simulink model "jav1"  (R2025b)
settings: Solver=VariableStepAuto  StartTime=0.0  StopTime=10.0  RelTol=1e-3
undefined symbols (not defined in the file): delta_pitch_saturation, g, I_treghet, K_drag, K_finne, Kd_pitch, Ki_altitude, Kp_altitude, Kp_pitch, L_aksial, m, T, theta0, theta_dot, theta_ff, theta_ref_saturation, v_x0, v_z0, x0, z0, z_ref
libraries: slpidlib x1
settings Model: Creator=Tobias Stenberg  LastModifiedBy=Tobias Stenberg

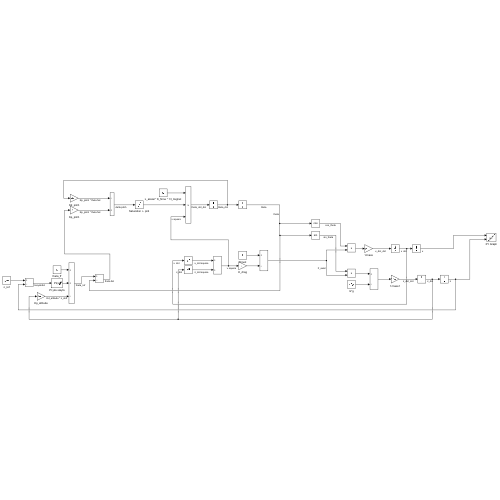
[thumbnail: Simulink's stored preview of the top-level diagram]
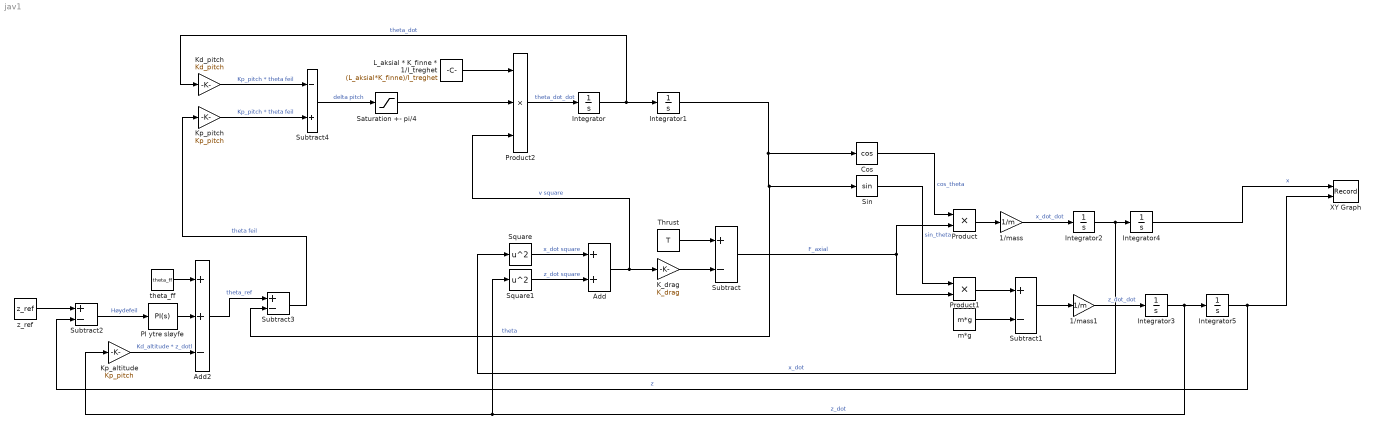
== system jav1 ==
  1/mass : Gain  Gain=1/m
  1/mass1 : Gain  Gain=1/m
  Add : Sum
  Add2 : Sum  Inputs=++-
  Cos : Trigonometry  Operator=cos
  Integrator : Integrator  InitialCondition=theta_dot
  Integrator1 : Integrator  InitialCondition=theta0
  Integrator2 : Integrator  InitialCondition=v_x0
  Integrator3 : Integrator  InitialCondition=v_z0
  Integrator4 : Integrator  InitialCondition=x0
  Integrator5 : Integrator  InitialCondition=z0
  K_drag : Gain  Gain=K_drag
  Kd_pitch : Gain  Gain=Kd_pitch
  Kp_altitude : Gain  Gain=Kp_pitch
  Kp_pitch : Gain  Gain=Kp_pitch
  L_aksial * K_finne * 1/I_treghet : Constant  Value=(L_aksial*K_finne)/I_treghet
  PI ytre sløyfe : slpidlib/PID Controller  Controller=PI  Form=Parallel  TimeDomain=Continuous-time  UseExternalTs=off  SampleTime=-1  IntegratorMethod=Forward Euler  FilterMethod=Forward Euler  ControllerParametersSource=internal  P=Kp_altitude  I=Ki_altitude  UseKiTs=off  D=0  UseExternalDerivativeSource=off  N=100  UseFilter=on  TunerSelectOption=Transfer Function Based (PID Tuner App)  ZeroCross=off  InitialConditionSource=internal  InitialConditionForIntegrator=0  InitialConditionForFilter=0  DifferentiatorICPrevScaledInput=0  ExternalReset=none  TrackingMode=off  Kt=1  LimitOutput=on  SatLimitsSource=internal  UpperSaturationLimit=theta_ref_saturation  LowerSaturationLimit=-theta_ref_saturation  LinearizeAsGain=on  AntiWindupMode=clamping  Kb=1  LimitIntegrator=off  UpperIntegratorSaturationLimit=inf  LowerIntegratorSaturationLimit=-inf  POutMin=[]  POutMax=[]  IOutMin=[]  IOutMax=[]  DOutMin=[]  DOutMax=[]  NOutMin=[]  NOutMax=[]  SumOutMin=[]  SumOutMax=[]  SaturationOutMin=[]  SaturationOutMax=[]  PParamMin=[]  PParamMax=[]  IParamMin=[]  IParamMax=[]  DParamMin=[]  DParamMax=[]  NParamMin=[]  NParamMax=[]  KbParamMin=[]  KbParamMax=[]  KtParamMin=[]  KtParamMax=[]  KbOutMin=[]  KbOutMax=[]  KtOutMin=[]  KtOutMax=[]  IntegratorOutMin=[]  IntegratorOutMax=[]  FilterOutMin=[]  FilterOutMax=[]  SumI1OutMin=[]  SumI1OutMax=[]  SumI2OutMin=[]  SumI2OutMax=[]  SumI3OutMin=[]  SumI3OutMax=[]  SumI4OutMin=[]  SumI4OutMax=[]  SumDOutMin=[]  SumDOutMax=[]  DifferentiatorOutMin=[]  DifferentiatorOutMax=[]  FilterDiffOutCoefMin=[]  FilterDiffOutCoefMax=[]  ReciprocalOutMin=[]  ReciprocalOutMax=[]  SumDenOutMin=[]  SumDenOutMax=[]  SumNumOutMin=[]  SumNumOutMax=[]  DivideOutMin=[]  DivideOutMax=[]  UdiffTsProdOutMin=[]  UdiffTsProdOutMax=[]  NTsProdOutMin=[]  NTsProdOutMax=[]  UintegralTsProdOutMin=[]  UintegralTsProdOutMax=[]  UngainTsProdOutMin=[]  UngainTsProdOutMax=[]  ClampingZeroOutDataTypeStr=Inherit: Inherit via back propagation  ClampingZeroOutMin=[]  ClampingZeroOutMax=[]  FilterDenConstantOutDataTypeStr=Inherit: Inherit via back propagation  FilterDenConstantOutMin=[]  FilterDenConstantOutMax=[]  PCopyOutDataTypeStr=Inherit: Inherit via back propagation  PCopyOutMin=[]  PCopyOutMax=[]  NCopyOutDataTypeStr=Inherit: Inherit via back propagation  NCopyOutMin=[]  NCopyOutMax=[]  IntegratorContinuousStateAttributes=''  IntegratorStateMustResolveToSignalObject=off  IntegratorRTWStateStorageClass=Auto  FilterContinuousStateAttributes=''  FilterStateMustResolveToSignalObject=off  FilterRTWStateStorageClass=Auto  ParallelPVariant=InternalParameters  IdealPVariant=Disabled  IVariant=InternalParameters  DVariant=Disabled  IntegratorVariant=Continuous  SatVariant=Enabled  AWVariant=ContClampingParallel  PCopyVariant=Disabled  TRVariant=Disabled  FdbkBlocksVariant=Forward  IdealPFdbkVariant=Disabled  SatFdbkVariant=Disabled  DerivativeFilterVariant=Disabled  NVariant=Disabled  NCopyVariant=Disabled_SignalSpec  FilterICVariant=Disabled  IntegratorICVariant=InternalICs  ExternalResetVariant=Disabled  TRSumVariant=Passthrough  SumFdbkVariant=Disabled  SumVariant=Sum_PI  TsampFilterVariant=InternalTs  TsampNgainVariant=Passthrough  TsampIntegralVariant=Disabled_SignalSpec  ExternalSaturationOutDataTypeStr=Inherit: Same as second input  DerivativeSourceVariant=Disabled  PreIntVariant=InternalPreInt
  Product : Product
  Product1 : Product
  Product2 : Product  Inputs=3
  Saturation +- pi/4 : Saturate  UpperLimit=delta_pitch_saturation  LowerLimit=-delta_pitch_saturation
  Sin : Trigonometry
  Square : Math  Operator=square
  Square1 : Math  Operator=square
  Subtract{,1..3} (4 alike) : Sum  Inputs=+-
  Subtract4 : Sum  Inputs=-+
  Thrust : Constant  Value=T
  XY Graph : Record  NumPorts=2.0  FileSettingsInternal="{\"entries\":[{\"content\":{\"excelSettings\":{\"content\":{},\"type\":\"Streamout.ExcelSettings\"},\"parquetSettings\":{\"content\":{},\"type\":\"Streamout.ParquetSettings\"}},\"type\":\"Streamout.FileSettingStorage\",\"uuid\":\"\"}],\"packageUris\":[\"http:\\/\\/schema.mathworks.com\\/mf0\\/streamout_blocks\\/R2020a\"],\"version\":\"1.0\"}"  FrameSettings=[0, 0]  Layout=[1 1]  SignalsInternal="{\"entries\":[{\"content\":{\"signals\":[{\"content\":{\"blockPath\":[],\"dimensions\":[1],\"domain\":\"\",\"lineColor\":\"#a2142f\",\"port\":1,\"signalID\":1,\"signalName\":\"x\"},\"type\":\"RecordBlkView.Signal\",\"uuid\":\"\"},{\"content\":{\"blockPath\":[],\"dimensions\":[1],\"domain\":\"\",\"lineColor\":\"#139fff\",\"plots\":[ 1 ],\"port\":2,\"signalID\":2,\"signalName\":\"z\"},\"type\":\"RecordBlkView.Signal\",\"uuid\":\"\"}]},\"type\":\"RecordBlkView.InputSignals\",\"uuid\":\"\"}],\"packageUris\":[\"http:\\/\\/schema.mathworks.com\\/mf0\\/streamout_blocks\\/R2020a\"],\"version\":\"1.0\"}"  CompatibilityTag=XY
  m*g : Constant  Value=m*g
  theta_ff : Constant  Value=theta_ff
  z_ref : Constant  Value=z_ref
  wires:
  Integrator/1 -> Kd_pitch/1, Integrator1/1  "theta_dot"
  Product2/1 -> Integrator/1  "theta_dot_dot"
  Integrator1/1 -> Subtract3/2, Sin/1, Cos/1  "theta"
  Square/1 -> Add/1  "x_dot square"
  Square1/1 -> Add/2  "z_dot square"
  Add/1 -> Product2/3, K_drag/1  "v square"
  K_drag/1 -> Subtract/2
  Thrust/1 -> Subtract/1
  Subtract/1 -> Product1/2, Product/2  "F_axial"
  Cos/1 -> Product/1  "cos_theta"
  Sin/1 -> Product1/1  "sin_theta"
  Product1/1 -> Subtract1/1
  m*g/1 -> Subtract1/2
  Subtract1/1 -> 1/mass1/1
  1/mass1/1 -> Integrator3/1  "z_dot_dot"
  Product/1 -> 1/mass/1
  1/mass/1 -> Integrator2/1  "x_dot_dot"
  Integrator2/1 -> Square/1, Integrator4/1  "x_dot"
  Integrator3/1 -> Square1/1, Kp_altitude/1, Integrator5/1  "z_dot"
  Integrator4/1 -> XY Graph/1  "x"
  Integrator5/1 -> Subtract2/2, XY Graph/2  "z"
  L_aksial * K_finne * 1/I_treghet/1 -> Product2/1
  z_ref/1 -> Subtract2/1
  Subtract2/1 -> PI ytre sløyfe/1  "Høydefeil"
  PI ytre sløyfe/1 -> Add2/2
  theta_ff/1 -> Add2/1
  Add2/1 -> Subtract3/1  "theta_ref"
  Subtract3/1 -> Kp_pitch/1  "theta feil"
  Saturation +- pi/4/1 -> Product2/2
  Subtract4/1 -> Saturation +- pi/4/1  "delta pitch"
  Kp_pitch/1 -> Subtract4/2  "Kp_pitch * theta feil"
  Kd_pitch/1 -> Subtract4/1  "Kp_pitch * theta feil"
  Kp_altitude/1 -> Add2/3  "Kd_altitude * z_dotl"
